simulink model "AM_RXTX_Audio_File"  (R2020b)
settings: Solver=VariableStepAuto  StartTime=0.0  StopTime=10  RelTol=1e-3
libraries: dspmlti4 x3, dspsnks4 x1, dspvision x1
settings Model: Creator=Guillaume  LastModifiedBy=Guillaume

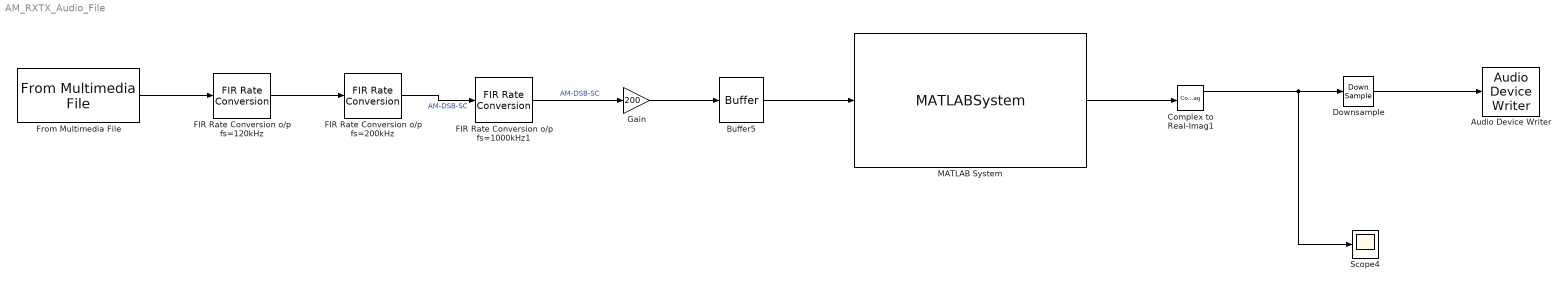
== system AM_RXTX_Audio_File ==
  Audio Device Writer : dspsnks4/Audio Device Writer  Driver=DirectSound  Device=Default  InheritSampleRate=on  SampleRate=44100  BitDepth=16-bit integer  BufferSize=4096  NumBuffers=10  DefaultOutputChannelMapping=on  OutputChannelMapping=1:2  OutputNumUnderrunSamples=off  DriverIdx=1  DeviceWarnFlag=''
  Buffer5 : Buffer  N=16384  OutputFrames=off
  Complex to Real-Imag1 : ComplexToRealImag
  Downsample : DownSample  N=21  RateOptions=Allow multirate processing
  FIR Rate Conversion o/p fs=1000kHz1 : dspmlti4/FIR Rate Conversion  FilterSource=Dialog parameters  L=5  h=firpm(100, [0 15e3 30e3 600e3/2]/(600e3/2), [1 1 0 0], [1 1],20)  M=1  FilterObject=Hm_firsrc  rateMode=Enforce single-rate processing  roundingMode=Floor  overflowMode=off  firstCoeffDataTypeStr=Inherit: Same word length as input  firstCoeffMin=[]  firstCoeffMax=[]  firstCoeffLastDataTypeStr=Inherit: Same word length as input  outputDataTypeStr=Inherit: Same as accumulator  outputMin=[]  outputMax=[]  outputLastDataTypeStr=Inherit: Same as accumulator
      settings: SourceProductBaseCode=DS
  FIR Rate Conversion o/p fs=120kHz : dspmlti4/FIR Rate Conversion  FilterSource=Dialog parameters  L=5  h=firpm(100, [0 15e3 24e3 240e3/2]/(240e3/2), [1 1 0 0], [1 1],20)  M=2  FilterObject=Hm_firsrc  rateMode=Enforce single-rate processing  roundingMode=Floor  overflowMode=off  firstCoeffDataTypeStr=Inherit: Same word length as input  firstCoeffMin=[]  firstCoeffMax=[]  firstCoeffLastDataTypeStr=Inherit: Same word length as input  outputDataTypeStr=Inherit: Same as accumulator  outputMin=[]  outputMax=[]  outputLastDataTypeStr=Inherit: Same as accumulator
      settings: SourceProductBaseCode=DS
  FIR Rate Conversion o/p fs=200kHz : dspmlti4/FIR Rate Conversion  FilterSource=Dialog parameters  L=5  h=firpm(100, [0 15e3 30e3 600e3/2]/(600e3/2), [1 1 0 0], [1 1],20)  M=3  FilterObject=Hm_firsrc  rateMode=Enforce single-rate processing  roundingMode=Floor  overflowMode=off  firstCoeffDataTypeStr=Inherit: Same word length as input  firstCoeffMin=[]  firstCoeffMax=[]  firstCoeffLastDataTypeStr=Inherit: Same word length as input  outputDataTypeStr=Inherit: Same as accumulator  outputMin=[]  outputMax=[]  outputLastDataTypeStr=Inherit: Same as accumulator
      settings: SourceProductBaseCode=DS
  From Multimedia File : dspvision/From Multimedia File  inputFilename=F:\Documents\MATLAB\LimeSDR\LimeSDR_Mini_Matlab_Github_2022\music1_mono48kHz.wav  readRange=[1 Inf]  loop=on  numPlays=inf  outputStreams=Audio only  videoDataType=single  audioDataType=single  inheritSampleTime=on  userDefinedSampleTime=1/30  noAudioOutput=off  isIntensityVideo=off  fourcc=RGB  colorVideoFormat=One multidimensional signal  outputEOF=off  dataOrg=Column-major  audioFrameSize=600  computeAudioFrameSize=off  outSamplingMode=Sample based
  Gain : Gain  Gain=200
  MATLAB System : MATLABSystem  System=limeSDR_Simulink_Wrapper_2022  enable_rx0=on  rx0_antenna=3  rx0_bandwidth=5  rx0_gain=20  rx_frequency=868e6  rx_samplerate=1e6  rx_timeout_ms=5000  rx_step_size=16384  enable_tx0=on  tx0_antenna=2  tx0_bandwidth=5  tx0_gain=30  tx_frequency=868e6  tx_samplerate=1e6  tx_timeout_ms=5000  tx_step_size=16384
      mask Type: limeSDR_Simulink_Wrapper_2022
      mask Display:
      | disp('LimeSDR mini');
      | port_label('input',1,'TX0 Samples');
      | port_label('output',1,'RX0 Samples');
  Scope4 : Scope
  wires:
  From Multimedia File/1 -> FIR Rate Conversion o/p fs=120kHz/1
  FIR Rate Conversion o/p fs=120kHz/1 -> FIR Rate Conversion o/p fs=200kHz/1
  MATLAB System/1 -> Complex to Real-Imag1/1
  FIR Rate Conversion o/p fs=200kHz/1 -> FIR Rate Conversion o/p fs=1000kHz1/1  "AM-DSB-SC"
  FIR Rate Conversion o/p fs=1000kHz1/1 -> Gain/1  "AM-DSB-SC"
  Gain/1 -> Buffer5/1
  Buffer5/1 -> MATLAB System/1
  Downsample/1 -> Audio Device Writer/1
  Complex to Real-Imag1/1 -> Scope4/1, Downsample/1
